simulink model "ACC_accel_MPC_adptv"  (R2024a)
settings: Solver=FixedStepAuto  StartTime=0  StopTime=100  FixedStep=.05  RelTol=1e-3
undefined symbols (not defined in the file or in its folder): act_t_delay, aero_const, Defined, delta_U_max, delta_U_min, driver_set_speed, Ego, Lane, m, matlabshared, output_accel_max, Qbar, Rbar, rho_ah_max, rho_ah_min, rho_vh_max, simStepSize, U_max, U_min, User
libraries: roadrunnerscenario x5, drivingscenarioandsensors x1, autolibshared x1
settings Model: PacingRate=10  Creator=darkh  LastModifiedBy=darkh
settings DataIOCC: ReturnWorkspaceOutputsName=sltest_internal_rrSimulationOutputVariable
settings OptimizationCC: ZeroExternalMemoryAtStartup=off  ZeroInternalMemoryAtStartup=off
settings DebuggingCC: AlgebraicLoopMsg=none
settings RTWCC: Description=Generate an RTMaps component embedding the model  SystemTargetFile=rtmaps.tlc  TemplateMakefile=rtmaps_default_tmf  PostCodeGenCommand=rtmaps_post_code_generation(buildInfo)  RetainRTWFile=on  TargetLang=C++  GPUComputeCapability=3.5
settings STFCustomTargetCC: TargetLangStandard=C++11 (ISO)  ModelReferenceCompliant=off  ConcurrentExecutionCompliant=on  CombineOutputUpdateFcns=on  CodeInterfacePackaging=C++ class  CPPClassGenCompliant=on  GRTInterface=off  UseToolchainInfoCompliant=off  SystemTargetFile=rtmaps.tlc
settings GRTTargetCC: TargetLangStandard=C++11 (ISO)  ModelReferenceCompliant=off  ParMdlRefBuildCompliant=off  CompOptLevelCompliant=off  MatFileLogging=off  CodeInterfacePackaging=C++ class  UseToolchainInfoCompliant=off
settings ConfigComp: CovSaveName=sltest_covdata  CovMetricSettings=dcmwe  CovEnableCumulative=off  CovSaveSingleToWorkspaceVar=on  CovSaveOutputData=off

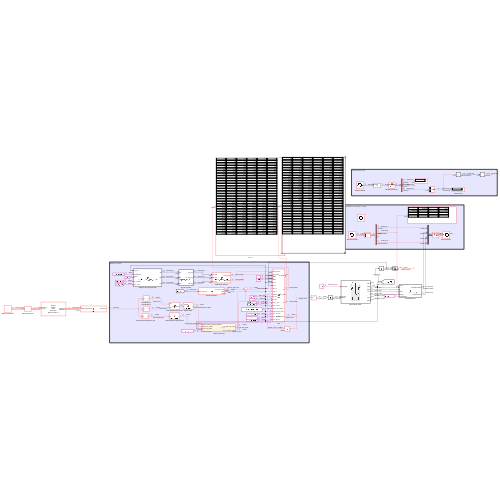
[thumbnail: Simulink's stored preview of the top-level diagram]
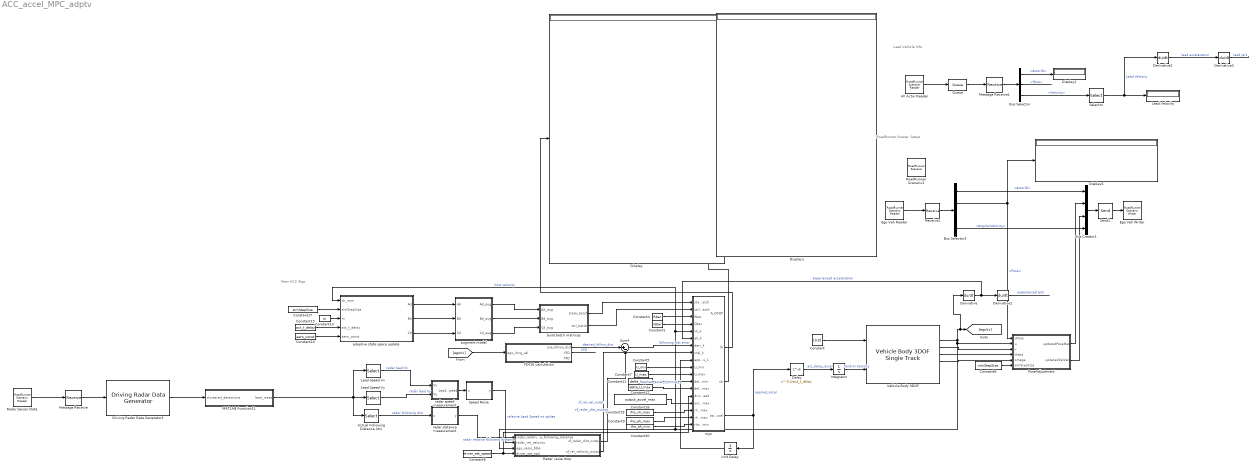
== system ACC_accel_MPC_adptv ==
  note: RoadRunner Scenar. Setup
  note: Lead Vehicle Info.
  note: Main ACC Algo
  Actual Following Distance (dx) : Selector  InputPortWidth=6  IndexOptions=Index vector (dialog)  Indices=[1]  OutputSizes=1
  All Actor Reader : roadrunnerscenario/RoadRunner Scenario Reader  TopicCategory=Actor  ActorCategory=All Types  ActionType=Path Following  EventType=User-Defined  TopicType=Actor Pose  VehicleType=Vehicle Specifications  UserDefinedAction=Action1  UserDefinedEvent=Event1  Filter=None  SensorTopic=Target Poses  LaneBoundaryOutputTopic=Ego-Lane  SensorID=1  SampleTime=simStepSize
  Bus Creator1 : BusCreator  Inputs=4  OutDataTypeStr=Bus: BusActorRuntime  NonVirtualBus=on
      settings: InheritFromInputs=off
  Bus Selector : BusSelector  OutputSignals=ActorID,Pose,Velocity
  Bus Selector3 : BusSelector  OutputSignals=ActorID,Pose,Velocity,AngularVelocity
  Constant : Constant  Value=[0,0]
  Constant1 : Constant  Value=Qbar
  Constant11 : Constant  Value=delta_U_min
  Constant12 : Constant  Value=delta_U_max
  Constant14 : Constant  Value=m
  Constant15 : Constant  Value=act_t_delay
  Constant16 : Constant  Value=aero_const
  Constant17 : Constant  Value=simStepSize
  Constant18 : Constant  Value=output_accel_max
  Constant19 : Constant  Value=rho_vh_max
  Constant20 : Constant  Value=rho_ah_min
  Constant4 : Constant  Value=Rbar
  Constant5 : Constant  Value=U_min
  Constant6 : Constant  Value=driver_set_speed
  Constant7 : Constant  Value=U_max
  Constant8 : Constant  Value=simStepSize
  Constant9 : Constant  Value=rho_ah_max
  Delay : Delay  DelayLength=0.2/act_t_delay
  Derivative{,1..3} (4 alike) : Derivative
  Display{,1..2,6} (4 alike) : Display
  Driving Radar Data Generator1 : drivingscenarioandsensors/Driving Radar Data Generator  SensorIndex=1  UpdateRate=20  MountingLocation=[ 3.4, 0, 0.2 ]  MountingAngles=[0 0 0]  HasElevation=off  HasRangeRate=on  HasNoise=off  HasFalseAlarms=off  HasOcclusion=on  MaxNumReportsSource=Property  MaxNumReports=50  TargetReportFormat=Clustered detections  DetectionCoordinates=Body  TrackCoordinates=Body  BusNameSource=Auto  BusName=BusDrivingRadarDataGenerator  AzimuthResolution=4  ElevationResolution=5  RangeResolution=2.5  RangeRateResolution=0.5  AzimuthBiasFraction=0.1  ElevationBiasFraction=0.1  RangeBiasFraction=0.05  RangeRateBiasFraction=0.05  FieldOfView=[ 20, 5 ]  RangeLimits=[ 0, 150 ]  RangeRateLimits=[ -100, 100 ]  DetectionProbability=0.9  FalseAlarmRate=1e-06  ReferenceRange=100  ReferenceRCS=0  CenterFrequency=77e9  FilterInitializationFcn=initcvekf  ConfirmationThreshold=[2 3]  DeletionThreshold=[5 5]  InitialSeedSource=Repeatable  InitialSeed=0  UsedSeed=matlabshared.tracking.internal.SimulinkUtilities.seedManager(gcb)  ProfilesSource=From Scenario Reader block  ProfilesParameters=driving.internal.ActorProfilesRadarParameters  ProfilesExpression=struct('ClassID',0,'Length',4.7,'Width',1.8,'Height',1.4,'OriginOffset',[-1.35 0 0],'RCSPattern',[10 10;10 10],'RCSAzimuthAngles',[-180 180],'RCSElevationAngles',[-90 90])
  Ego Veh Reader : roadrunnerscenario/RoadRunner Scenario Reader  TopicCategory=Actor  ActorCategory=All Types  ActionType=Path Following  EventType=User-Defined  TopicType=Actor Pose  VehicleType=Vehicle Specifications  UserDefinedAction=Action1  UserDefinedEvent=Event1  Filter=Self  SensorTopic=Target Poses  LaneBoundaryOutputTopic=Ego-Lane  SensorID=1  SampleTime=simStepSize
  Ego Veh Writer : roadrunnerscenario/RoadRunner Scenario Writer  TopicCategory=Actor  ActorCategory=All Types  EventType=Action Complete  UserDefinedEvent=Event1  VehicleType=Vehicle Pose  TopicType=Actor Pose
  FDCW calculation : MATLAB Function  TreatAsAtomicUnit=on
  Integrator : Integrator
  Lead Speed Vx : Selector  InputPortWidth=6  IndexOptions=Index vector (dialog)  Indices=4  OutputSizes=1
  Lead Speed Vy : Selector  InputPortWidth=6  IndexOptions=Index vector (dialog)  Indices=5  OutputSizes=1
  Lead Velocity : Display
  MATLAB Function11 : MATLAB Function  TreatAsAtomicUnit=on
  Message Receive : Receive  InputPortMessageModes=m  UseInternalQueue=off
  Message Receive1 : Receive  InputPortMessageModes=m
  PoseAdjustment : MATLAB Function  TreatAsAtomicUnit=on
  Queue : Queue  InputPortMessageModes=m  OutputPortMessageModes=m  OverwriteOldest=on  Capacity=16  QueueType=LIFO
  Radar Sensor Data : roadrunnerscenario/RoadRunner Scenario Reader  TopicCategory=Sensor  ActorCategory=All Types  ActionType=Path Following  EventType=User-Defined  TopicType=Actor Specifications  VehicleType=Vehicle Specifications  UserDefinedAction=Action1  UserDefinedEvent=Event1  Filter=Self  SensorTopic=Target Poses  LaneBoundaryOutputTopic=Ego-Lane  SensorID=1  SampleTime=simStepSize
  Radar value drop : Stateflow chart  TreatAsAtomicUnit=on
  Receive1 : Receive  InputPortMessageModes=m  UseInternalQueue=off  QueueOverwriting=on  QueueLength=1  QueueType=LIFO
  RoadRunner Scenario1 : roadrunnerscenario/RoadRunner Scenario  UserDefinedActions={}  UserDefinedEvents={}
  Selector : Selector  InputPortWidth=3  IndexOptions=Index vector (dialog)  Indices=[2]  OutputSizes=1
  Send1 : Send  OutputPortMessageModes=m
  Speed Noise : MATLAB Function  TreatAsAtomicUnit=on
  Sum4 : Sum  Inputs=|+-
  Unit Delay : UnitDelay  SampleTime=-1  HasFrameUpgradeWarning=on
  "Vehicle Body 3DOF " : autolibshared/Vehicle Body 3DOF Single Track  trackMode=Dual  inputMode=External longitudinal velocity  frontSteerMode=on  rearSteerMode=off  windMode=off  muMode=off  extFMode=off  extMMode=off  htchFMode=off  htchMMode=off  extXo=off  extpsio=off  extxdoto=off  extro=off  extYo=off  extTamb=off  extydoto=off  aMode=2  NF=2  NR=2  m=m  a=1.5569  b=1.5371  h=0.18903  dh=1  hh=0.2  X_o=0  xdot_o=0  CalphaMode=off  sigmaMode=on  d=0  hl=0  w=[1.4,1.4]  Cy_f=40000  Cy_r=40000  sigma_f=.1  sigma_r=.1  alpha_f_brk=[-.1 .1]  Cy_f_data=[-9e3 9e3]  alpha_r_brk=[-.1 .1]  Cy_r_data=[-9e3 9e3]  Y_o=0  ydot_o=0  Izz=2066  psi_o=0  r_o=0  Af=2.73  Cd=.30356  Cl=.1  Cpm=.1  beta_w=[0 0.01:0.01:0.3]  Cs=[0 0.01:0.01:0.3]  Cym=[0 1e-6:0.01:0.3]  Pabs=101325  Tair=273  g=9.81  mu=1  xdot_tol=.01  Fznom=5000  Fxtire_sat=7e4  Fytire_sat=7e4  longOff=0  latOff=0  vertOff=0  wrapAng=off
  adaptive state space update : MATLAB Function  TreatAsAtomicUnit=on
  augment model : MATLAB Function  TreatAsAtomicUnit=on
  build batch matrices : MATLAB Function  TreatAsAtomicUnit=on  SystemSampleTime=simStepSize
  mpc : MATLAB Function  TreatAsAtomicUnit=on  SystemSampleTime=simStepSize
  radar distance measurement : MATLAB Function  TreatAsAtomicUnit=on
  radar speed measurement : MATLAB Function  TreatAsAtomicUnit=on
  wires:
  Bus Selector3/4 -> Bus Creator1/4  "<AngularVelocity>"
  Bus Creator1/1 -> Send1/1
  Bus Selector3/1 -> Bus Creator1/1  "<ActorID>"
  Receive1/1 -> Bus Selector3/1
  Send1/1 -> Ego Veh Writer/1
  Ego Veh Reader/1 -> Receive1/1
  Bus Selector3/2 -> Display6/1, PoseAdjustment/1(cPose)  "<Pose>"
  PoseAdjustment/1(updatedPoseMat) -> Bus Creator1/2
  "Vehicle Body 3DOF "/2 -> PoseAdjustment/2(u), Radar value drop/3(ego_veloc_fdbk), adaptive state space update/1(vh_nom), mpc/5(vh_k), Derivative/1, [egoVx]  "host velocity"
  Radar Sensor Data/1 -> Message Receive/1
  Message Receive/1 -> Driving Radar Data Generator1/1
  Driving Radar Data Generator1/1 -> MATLAB Function11/1(clustered_detections)
  PoseAdjustment/2(updatedVelVec) -> Bus Creator1/3
  Integrator/1 -> "Vehicle Body 3DOF "/2  "Control Velocity"
  Constant/1 -> "Vehicle Body 3DOF "/1
  Sum4/1 -> mpc/7(derr_k)  "following dist error"
  Speed Noise/1(y) -> Radar value drop/2(radar_rel_velocity)  "relative Lead Speed no spikes"
  Lead Speed Vx/1 -> radar speed measurement/1(Vx)  "radar lead Vx"
  [egoVx] -> FDCW calculation/1(ego_long_vel)
  FDCW calculation/1(ave_follow_dist) -> Sum4/1  "desired_follow_dist"
  MATLAB Function11/1(lead_meas) -> Actual Following Distance (dx)/1, Lead Speed Vx/1, Lead Speed Vy/1
  radar distance measurement/1(y) -> Radar value drop/1(radar_relative_following_distance)  "radar relative following distance"
  Lead Speed Vy/1 -> radar speed measurement/2(Vy)  "radar lead Vy"
  radar speed measurement/1(LeadSpeed) -> Speed Noise/1(u)
  FDCW calculation/2(CFD) -> ?  "CFD"
  Actual Following Distance (dx)/1 -> radar distance measurement/1(u)  "radar following dist"
  Derivative/1 -> mpc/6(ah_k), Derivative1/1  "experienced acceleration"
  Derivative1/1 -> ?  "experienced jerk"
  Constant4/1 -> mpc/3(Rbar)
  Radar value drop/1(sf_radar_dist_output) -> Sum4/2  "sf_radar_dist_output"
  Constant6/1 -> mpc/14(driver_set_speed), Radar value drop/4(driver_set_spd)
  Radar value drop/2(sf_rel_velocity_output) -> mpc/8(vrel_k)  "sf_rel_vel_outpt"
  Unit Delay/1 -> mpc/9(applied_accel_k_minus_1)  "applied_accel_k_minus_1"
  Constant5/1 -> mpc/10(U_min)
  Constant7/1 -> mpc/11(U_max)
  Constant8/1 -> PoseAdjustment/6(simStepSize)
  Constant9/1 -> mpc/17(rho_ah_max)
  Constant11/1 -> mpc/12(del_U_min)
  Constant12/1 -> mpc/13(del_U_max)
  "Vehicle Body 3DOF "/4 -> PoseAdjustment/4(theta)
  Constant1/1 -> mpc/4(Qbar)
  "Vehicle Body 3DOF "/5 -> PoseAdjustment/5(omega)
  "Vehicle Body 3DOF "/3 -> PoseAdjustment/3(v)
  mpc/4(applied_accel) -> Delay/1, Unit Delay/1  "applied_accel"
  Constant14/1 -> adaptive state space update/3(m)
  Constant15/1 -> adaptive state space update/4(act_t_delay)
  Constant16/1 -> adaptive state space update/5(aero_const)
  Constant17/1 -> adaptive state space update/2(simStepSize)
  augment model/3(Cd_aug) -> build batch matrices/3(Cd_aug)
  augment model/2(Bd_aug) -> build batch matrices/2(Bd_aug)
  augment model/1(Ad_aug) -> build batch matrices/1(Ad_aug)
  adaptive state space update/1(Ad) -> augment model/1(Ad)
  adaptive state space update/2(Bd) -> augment model/2(Bd)
  adaptive state space update/3(Cd) -> augment model/3(Cd)
  Delay/1 -> Integrator/1  "act_delay_accel"
  build batch matrices/1(state_batch) -> mpc/1(state_batch)
  build batch matrices/2(ctrl_batch) -> mpc/2(ctrl_batch)
  Constant18/1 -> mpc/15(output_accel_max)
  Constant19/1 -> mpc/16(rho_vh_max)
  Constant20/1 -> mpc/18(rho_ah_min)
  All Actor Reader/1 -> Queue/1
  Queue/1 -> Message Receive1/1
  Message Receive1/1 -> Bus Selector/1
  Bus Selector/1 -> Display2/1  "<ActorID>"
  Bus Selector/2 -> ?  "<Pose>"
  Bus Selector/3 -> Selector/1  "<Velocity>"
  Selector/1 -> Derivative2/1, Lead Velocity/1  "Lead Velocity"
  Derivative2/1 -> Derivative3/1  "lead acceleration"
  Derivative3/1 -> ?  "lead jerk"
  mpc/2(lb) -> Display/1
  mpc/3(ub) -> Display1/1

== matlab function ACC_accel_MPC_adptv/build batch matrices ==
  data: state_batch output; Ad_aug input; Bd_aug input; Cd_aug input; ctrl_batch output
function [state_batch,ctrl_batch] = batch_matrix_build(Ad_aug,Bd_aug,Cd_aug)
[ny1,ny2] = size(Cd_aug);
[~,nu] = size(Bd_aug);

N=20;

% Building batch matrices for MPC prediction of output states
% batch matrix for state vector
state_batch = zeros(N*ny1, ny2);
for i = 1:N
    state_batch((i-1)*ny1+1 : i*ny1, :) = Cd_aug*(Ad_aug^i);
end

% Batch matrix for control vector
ctrl_batch = zeros(N*ny1, N*nu); % pre-allocate, fixed size

Apow = eye(size(Ad_aug)); % A^0
for i = 1:N
    % first column block for row i
    ctrl_batch((i-1)*ny1+(1:ny1), 1:nu) = Cd_aug*Apow*Bd_aug;
    % copy to the right for j = 2…i
    col = nu; % offset for next column
    Apow_j = Apow;
    for j = 2:i
        Apow_j = Apow_j / Ad_aug; % A^(i-j) (cheaper than repeated power)
        ctrl_batch((i-1)*ny1+(1:ny1), (j-1)*nu+(1:nu)) = Cd_aug*Apow_j*Bd_aug;
        col = col + nu;
    end
    Apow = Apow*Ad_aug; % advance A^i
end

== matlab function ACC_accel_MPC_adptv/PoseAdjustment ==
  data: cPose input; u input; updatedPoseMat output; v input; theta input; omega input; updatedVelVec output; simStepSize input
function [updatedPoseMat, updatedVelVec] = RRPoseAdjustment(cPose, u, v, theta, omega, simStepSize)
    thetad = theta + omega*simStepSize;
    xd = (u*cos(theta) - v*sin(theta))*simStepSize;
    yd = (u*sin(theta) + v*cos(theta))*simStepSize;
    pose_mat = [cos(-thetad) -sin(-thetad) 0 (yd+cPose(1,4)); sin(-thetad) cos(-thetad) 0 (xd+cPose(2,4)); 0 0 1 0; 0 0 0 1];
    updatedPoseMat = pose_mat;
    updatedVelVec = [u*sin(theta) + v*cos(theta), u*cos(theta) - v*sin(theta), 0];
    return;
end

== matlab function ACC_accel_MPC_adptv/radar distance measurement ==
  data: u input; y output
function y = removeSpikes(u)

    persistent buffer;
    persistent bufferIndex;
    threshold = 2;
    % windowSize = 15;
    windowSize = 5;
    
    if isempty(buffer)
        buffer = zeros(1, windowSize);
        bufferIndex = 1;
    end
    
    % Update buffer with new value
    buffer(bufferIndex) = u;
    bufferIndex = mod(bufferIndex, windowSize) + 1;
    
    % Calculate the median of the buffer
    medVal = median(buffer);
    
    % Detect and remove spikes
    if abs(u - medVal) > threshold
        y = medVal; % Replace spike with the median value
    else
        y = u; % Keep the original value if it's not a spike
    end
end

== matlab function ACC_accel_MPC_adptv/radar speed measurement ==
  data: Vx input; LeadSpeed output; Vy input
function LeadSpeed = fcn(Vx, Vy)

if Vx == 0 && Vy == 0 
    Vx = 0.01;
    Vy = 0.01;
elseif Vy == 0
    Vy = 0.01;
elseif Vx == 0
    Vx = 0.01;
end

if Vx <= 0
    LeadSpeed = -sqrt(Vx^2 + Vy^2);
else
    LeadSpeed = sqrt(Vx^2 + Vy^2);
end

== matlab function ACC_accel_MPC_adptv/Speed Noise ==
  settings: updateMethod=DISCRETE
  data: u input; y output
function y = removeSpikes(u)
    % removeSpikes - Removes spikes from a scalar signal based on a threshold
    %
    % Inputs:
    %    u - The input signal (scalar)
    %    threshold - The threshold value to detect spikes
    %    windowSize - The size of the window for calculating the median
    %
    % Outputs:
    %    y - The filtered signal with spikes removed

    % Declare persistent variables to store past values
    persistent buffer;
    persistent bufferIndex;
    threshold = 2;
    % windowSize = 15;
    windowSize = 5;

    
    if isempty(buffer)
        buffer = zeros(1, windowSize);
        bufferIndex = 1;
    end
    
    % Update buffer with new value
    buffer(bufferIndex) = u;
    bufferIndex = mod(bufferIndex, windowSize) + 1;
    
    % Calculate the median of the buffer
    medVal = median(buffer);
    
    % Detect and remove spikes
    if abs(u - medVal) > threshold
        y = medVal; % Replace spike with the median value
    else
        y = u; % Keep the original value if it's not a spike
    end
end

== matlab function ACC_accel_MPC_adptv/MATLAB Function11 ==
  data: clustered_detections input Bus: BusRadar; lead_meas output double
function lead_meas = fcn(clustered_detections)

lead_det = clustered_detections.Detections(1);
lead_meas = lead_det.Measurement;

% relative_dist = sqrt(lead_det.Measurement(1)^2 + lead_det.Measurement(2)^2); % rel_dist = sqrt(x^2+y^2)
% relative_speed = sqrt(lead_det.Measurement(4)^2 + lead_det.Measurement(5)^2);
end

== matlab function ACC_accel_MPC_adptv/FDCW calculation ==
  settings: updateMethod=DISCRETE
  data: ego_long_vel input; ave_follow_dist output; CFD output; FFD output
% Function to determine the closest (CFD) and furthest follow distance (FFD) for the
% ego vehicle relative to the lead vehicle given the ego vehicle's current
% velocity

% This function outputs the middle distance value between the CFD and FFD
% and those values respectively as well

function [ave_follow_dist, CFD, FFD] = fcn(ego_long_vel)
    persistent dist_history window_size smoothing_weights
    
    % Initialize (first call only)
    if isempty(dist_history)
        window_size = 5;  % Number of past samples
        dist_history = zeros(1, window_size);
        
        % Define and normalize weights (e.g., linear decay)
        smoothing_weights = linspace(1, 0.5, window_size);  % Weights from 1.0 to 0.5
        smoothing_weights = smoothing_weights / sum(smoothing_weights);  % Normalize
    end
    ego_long_vel_mph = ego_long_vel*2.23694;
    
    if ego_long_vel_mph > 0 && ego_long_vel_mph < 20
        CFD = 2.8*ego_long_vel_mph^0.45+8;
        FFD = 100-0.2*(20-ego_long_vel_mph)^2;
    elseif ego_long_vel_mph <= 0
        CFD = 8;
        FFD = 100-0.2*(20)^2;
    else
        CFD = 2.8*ego_long_vel_mph^0.45+8;
        FFD = 100;
    end
    AveFollowDist_Gain = 3;


    % --- Update history buffer ---
    dist_history = [ ((AveFollowDist_Gain-1)*CFD + FFD)/AveFollowDist_Gain , dist_history(1:end-1)];  % FIFO

    % --- Smoothed average (weighted, normalized) ---
    smoothed_ave_dist = sum(dist_history .* smoothing_weights);
    
    % --- Clamp to CFD/FFD bounds ---
    ave_follow_dist = min(max(smoothed_ave_dist, CFD), FFD);
end

== matlab function ACC_accel_MPC_adptv/adaptive state space update ==
  data: vh_nom input; simStepSize input; Ad output; m input; act_t_delay input; aero_const input; Bd output; Cd output
function [Ad,Bd,Cd] = adaptive_state_space_model(vh_nom, simStepSize, m, act_t_delay, aero_const)
% multiplying A matrix term with current vehicle velocity vh_nom to update
% state space model for adaptive MPC
Ac = [-aero_const*vh_nom/m,1,0,0; 0, -1/act_t_delay, 0,0; 0,0,0,-1; aero_const*vh_nom/m,-1,0,0];
Bc = [0;1/act_t_delay;0;0];

% Using Euler discretization to obtain the discrete time matrices from the continuous time system
Ad = eye(4) + Ac.*simStepSize;
Bd = Bc.*simStepSize;
Cd = eye(4);

== matlab function ACC_accel_MPC_adptv/mpc ==
  data: A_OSQP output; lb output; ub output; state_batch input; ctrl_batch input; Rbar input; Qbar input; applied_accel output; vh_k input; ah_k input; derr_k input; vrel_k input; applied_accel_k_minus_1 input; U_min input; U_max input; del_U_min input; del_U_max input; driver_set_speed input; output_accel_max input; rho_vh_max input; rho_ah_max input; rho_ah_min input
function [A_OSQP, lb, ub, applied_accel] = mpc(state_batch, ctrl_batch, Rbar, Qbar, vh_k, ah_k, derr_k, vrel_k, applied_accel_k_minus_1, U_min, U_max, del_U_min, del_U_max, driver_set_speed, output_accel_max, rho_vh_max, rho_ah_max, rho_ah_min)
% Defining MPC and system variables
N = 20;
num_constrained_outpts = 2;
num_ctrl = 1;

state_vec_curr = [vh_k, ah_k, derr_k, vrel_k, applied_accel_k_minus_1]';

%% Building the batch matrices with matrix mask T_v_a which would give full predicted vector with just the host velocity and host acceleration values
v_a_mask = kron(eye(N),[1,0,0,0;0,1,0,0]);
state_batch_v_a = v_a_mask*state_batch;
ctrl_batch_v_a = v_a_mask*ctrl_batch;

v_mask = kron(eye(N),[1,0,0,0]);
state_batch_v = v_mask*state_batch;
ctrl_batch_v = v_mask*ctrl_batch;

a_mask = kron(eye(N),[0,1,0,0]);
state_batch_a = a_mask*state_batch;
ctrl_batch_a = a_mask*ctrl_batch;

L = zeros(N*2, N);
for i = 1:N
    L(i*2:i*2, i:i) = 1;
end

W = zeros(N*2,N);
for i = 1:N
    W(i*2-1:i*2-1, i:i) = 1;
end

%% Building hessian, H, and f matrices for quadratic cost functional
H = blkdiag(2*(ctrl_batch'*Qbar*ctrl_batch + Rbar), 2*rho_vh_max*eye(N), 2*rho_ah_max*eye(N), 2*rho_ah_min*eye(N));
f = [2*ctrl_batch'*Qbar*state_batch*state_vec_curr; zeros(N,1); zeros(N,1); zeros(N,1)];
H = (H+H.')/2 + 1e-8*eye(size(H)); % tiny regulariser to ensure positive-definite

% H = 2*(ctrl_batch' * Qbar * ctrl_batch + Rbar); % symmetric Hessian without slack variables penalty
% f = 2*(ctrl_batch' * Qbar * state_batch * state_vec_curr); 

% Code gen for the OSQP solver since it needs to be defined as extrinsic function in MATLAB
coder.extrinsic('OSQP_MPC_helper');

persistent del_Uopt_k_minus_1 opt_qp_vec_k_minus_1 % defining persistent variable to keep track of computed optimal control signal from previous iteration
if isempty(del_Uopt_k_minus_1)
    % del_Uopt_k_minus_1 = [0,0,0,0,0,0,0,0,0,0]'; % for N = 10
    % del_Uopt_k_minus_1 = [0,0,0,0,0,0,0,0,0,0,0,0,0,0,0,0,0,0,0,0]'; % for N = 20
    % opt_qp_vec_k_minus_1 = zeros(80,1);
    
    del_Uopt_k_minus_1 = zeros(N,1);
    opt_qp_vec_k_minus_1 = zeros(4*N,1);

    % % Initializing the OSQP MPC solver with empty matrices once at
    % % beginning of program then updating the rest of the timesteps
    % MPC_OSQP_Instance = osqp;
    % % Initializing setup with empty constraints as well just for size allocation; Sizes must match those matrices used in the update function
    % MPC_OSQP_Instance.setup(H, f, ones(7*N, 4*N), zeros(7*N,1), zeros(7*N,1), 'warm_start', true, 'verbose', false); % .setup(P,q,A,lb,ub)
    OSQP_MPC_helper(N,num_ctrl,H,f,ones(9*N, 4*N), zeros(9*N,1), ones(9*N,1)); % Setup step
end

%% Defining the control input limits on delta_u based on limits on u

% Determining U(k-1) from the previous control signal u(k-1) and the previous full predicted control signal delta_Uopt(k-1)
Ubar_k_minus_1 = zeros(N*num_ctrl, 1); % Initializing
Ubar_k_minus_1(1:num_ctrl,:) = applied_accel_k_minus_1; % Populating the first control vector in Uopt(k-1) as u(k-1) = [accel_app(k-1)]'

for i = 1:N-1
    Ubar_k_minus_1(i*num_ctrl+1 : (i+1)*num_ctrl, :) = Ubar_k_minus_1((i-1)*num_ctrl+1 : i*num_ctrl, :) + del_Uopt_k_minus_1(i*num_ctrl+1 : (i+1)*num_ctrl, :); % performing u(k) = u(k-1) + delta_u(k-1) for all elements to populate Uopt(k-1)
end

% Defining the maximum and minimum output limits to be applied to the full prediction vector since the driver set speed may change
Y_max = zeros(N*num_constrained_outpts, 1);
Y_min = zeros(N*num_constrained_outpts, 1);
for i = 1:N
    Y_max((i-1)*num_constrained_outpts + 1: i*num_constrained_outpts,:) = [driver_set_speed; output_accel_max];
    Y_min((i-1)*num_constrained_outpts + 1: i*num_constrained_outpts,:) = [0.0; -output_accel_max];
end

%% Constraints
% % Constraints on input: applied acceleration
% A_ineq_input = [eye(N*num_ctrl), zeros(N, N), zeros(N,N), zeros(N,N); -eye(N*num_ctrl), zeros(N, N), zeros(N,N), zeros(N,N)];
% b_ineq_input = [U_max - Ubar_k_minus_1; -U_min + Ubar_k_minus_1];
% 
% % Constraints on outputs: vh and ah, derr and vrel are unconstrained
% A_ineq_outpt = [ctrl_batch_v_a, -W, -L, zeros(N*2,N); -ctrl_batch_v_a, zeros(N*2, N), zeros(N*2, N), -L];
% b_ineq_outpt = [Y_max - state_batch_v_a*state_vec_curr; -Y_min + state_batch_v_a*state_vec_curr];

%% Compiling both input and output constraints into single A*z < b format
% A_qp = [A_ineq_input; A_ineq_outpt];
% b_qp = [b_ineq_input; b_ineq_outpt]; 

%% New constraint formulation for OSQP
lb = [-3.5*ones(N,1)-Ubar_k_minus_1; -0.25*ones(N,1); zeros(3*N,1); -10000*ones(2*N,1); -10000*ones(2*N,1)];
ub = [3.5*ones(N,1)-Ubar_k_minus_1; 0.25*ones(N,1); 10000*ones(3*N,1); driver_set_speed*ones(N,1)-state_batch_v*state_vec_curr; state_batch_v*state_vec_curr; output_accel_max*ones(N,1)-state_batch_a*state_vec_curr; output_accel_max*ones(N,1)+state_batch_a*state_vec_curr];
A_OSQP = [eye(N), zeros(N,3*N); eye(N), zeros(N,3*N); zeros(N,N), eye(N), zeros(N,2*N); zeros(N,2*N), eye(N), zeros(N,N); zeros(N,3*N), eye(N); ctrl_batch_v, -eye(N), zeros(N, 2*N); -ctrl_batch_v, zeros(N, 3*N); ctrl_batch_a, zeros(N,N), -eye(N), zeros(N,N); -ctrl_batch_a, zeros(N,2*N), -eye(N)];

% % Compiling all input and output (including input deviation) constraints in lb <= A*z <= ub
% A_osqp = [A_ineq_input; A_ineq_outpt; eye(N), zeros(N,N), zeros(N,N), zeros(N,N)];
% lb_osqp = [-1000000000*ones(6*N, 1); -0.25*ones(N,1)]; 
% ub_osqp = [b_ineq_input; b_ineq_outpt; 0.25*ones(N,1)];

%% Running the optimizer
%% quadprog is used to solve the optimization problem
% options = optimoptions('quadprog','Algorithm','active-set'); % options for quadprog
% opt_qp_vec = quadprog(H,f,A_qp,b_qp,[],[],del_U_min,del_U_max,opt_qp_vec_k_minus_1,options); % includes constraints on delta_u here
% delta_Uopt_qp = opt_qp_vec(1:N*num_ctrl,:); % extracting predicted optimized control signal without the slack variables
% opt_qp_vec_k_minus_1 = opt_qp_vec; % To be used in the next instance of quadprog
% del_Uopt_k_minus_1 = delta_Uopt_qp; % saving computed control signal for optimal delta U (over prediction horizon) for use in next iteration; becomes next delta_Uopt(k-1)
% delta_u_apply = delta_Uopt_qp(1:num_ctrl,:); % nu = number of inputs; receding horizon so only selecting the first control vector in collection to apply to plant

%% OSQP solver update and control signal step
delta_Uopt_OSQP = zeros(N,1);
delta_Uopt_OSQP(:,:) = OSQP_MPC_helper(N,num_ctrl,H,f,A_OSQP,lb,ub); % Update step through extrinsic function in MATLAB
del_Uopt_k_minus_1 = delta_Uopt_OSQP; % saving computed control signal for optimal delta U (over prediction horizon) for use in next iteration; becomes next delta_Uopt(k-1)
delta_u_apply = delta_Uopt_OSQP(1);

applied_accel = applied_accel_k_minus_1 + delta_u_apply; % Adding to previous control input since state space model is augmented to determine delta_u

== stateflow chart ACC_accel_MPC_adptv/Radar value drop ==
  state Radar_State_Lead_Veh_Present_and_Detected
    sf_radar_dist_output = radar_relative_following_distance;
    % sf_radar_dist_output = smooth_switch(sf_radar_dist_output, radar_relative_following_distance, 0.05, 2);
    sf_rel_velocity_output = radar_rel_velocity;
    %sf_rel_velocity_output = smooth_switch(sf_rel_velocity_output, radar_rel_velocity, 0.05, 1);
  state Output_Spoof_To_Keep_Moving
    % sf_radar_dist_output = 150;
    sf_radar_dist_output = smooth_switch(sf_radar_dist_output, 150, 0.05, 2);
    set_spd_err = driver_set_spd - ego_veloc_fdbk;
    % sf_rel_velocity_output = set_spd_err;
    sf_rel_velocity_output = smooth_switch(sf_rel_velocity_output, set_spd_err, 0.05, 5);
  (default) -> Radar_State_Lead_Veh_Present_and_Detected : {sf_radar_dist_output = radar_relative_following_distance;
      | sf_rel_velocity_output = radar_rel_velocity;}
  Radar_State_Lead_Veh_Present_and_Detected -> Output_Spoof_To_Keep_Moving : [radar_relative_following_distance == 0 && radar_rel_velocity < 0.9]
  Output_Spoof_To_Keep_Moving -> Radar_State_Lead_Veh_Present_and_Detected : [radar_relative_following_distance > 0]
  data: prev_val function_input; curr_val function_input; dt function_input; tau function_input; filtered_val function_output; radar_relative_following_distance input; sf_radar_dist_output output; radar_rel_velocity input; ego_veloc_fdbk input; sf_rel_velocity_output output; driver_set_spd input; set_spd_err local
  function filtered_val = smooth_switch(prev_val, curr_val, dt, tau):
    | function filtered_val = smooth_switch(prev_val, curr_val, dt, tau)
    | % Smooth transition from prev_val toward curr_val
    | % dt  = sample time [s]; equal to system sample time of 0.05s currently
    | % tau = time constant [s] (0.3–1.0 typical)
    | 
    | if isempty(prev_val)
    |     prev_val = 0;
    | end
    | 
    | alpha = exp(-dt/tau);
    | filtered_val = alpha*prev_val + (1-alpha)*curr_val;
    | end

== matlab function ACC_accel_MPC_adptv/augment model ==
  data: Ad input; Ad_aug output; Bd input; Cd input; Bd_aug output; Cd_aug output
function [Ad_aug,Bd_aug,Cd_aug] = augment_ss_model(Ad,Bd,Cd)
[num_states,~] = size(Ad); % number of states in unaugmented system model
[~,num_ctrl] = size(Bd); % number of control inputs to system
[num_outpts,~] = size(Cd); % number of outputs from system

% Augmenting the State space model to have control vector delta_u and new state vec [x(k)', u(k-1)]' and output vec y(k) = x(k) 
Ad_aug = [Ad, Bd; zeros([num_ctrl num_states]), eye(num_ctrl)];
Bd_aug = [Bd; eye(num_ctrl)];
Cd_aug = [Cd, zeros([num_outpts num_ctrl])];
